simulink model "myrobot"  (R2019b)
settings: Solver=FixedStepAuto  StartTime=0.0  StopTime=2  FixedStep=0.001  MaxStep=0.005  RelTol=1e-3
undefined symbols (not defined in the file or in its folder): X, Y, Z
libraries: sm_lib x17, nesl_utility x13, robotmaniplib x4, simulink x2
(part 1 of 7)
settings Model: Creator=jglee  LastModifiedBy=jglee
settings SolverCC: AlgebraicLoopSolver=LineSearch

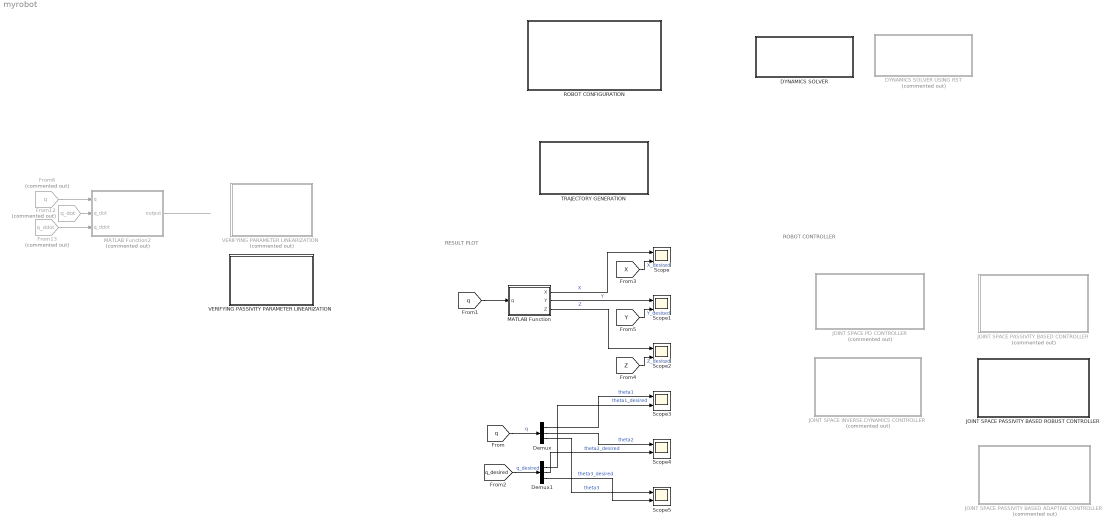
== system myrobot ==
  note: ROBOT CONTROLLER
  note: RESULT PLOT
  DYNAMICS SOLVER : Subsystem
  DYNAMICS SOLVER USING RST : Subsystem  Commented=on
  Demux : Demux  Outputs=3
  Demux1 : Demux  Outputs=3
  From12 : From  Commented=on  GotoTag=q_dot  TagVisibility=global
  From13 : From  Commented=on  GotoTag=q_ddot  TagVisibility=global
  From6 : From  Commented=on  GotoTag=q  TagVisibility=global
  JOINT SPACE INVERSE DYNAMICS CONTROLLER : Subsystem  Commented=on
  JOINT SPACE PASSIVITY BASED ADAPTIVE CONTROLLER : Subsystem  Commented=on
  JOINT SPACE PASSIVITY BASED CONTROLLER : Subsystem  Commented=on
  JOINT SPACE PASSIVITY BASED ROBUST CONTROLLER : Subsystem
  JOINT SPACE PD CONTROLLER : Subsystem  Commented=on
  MATLAB Function : MATLAB Function  TreatAsAtomicUnit=on
  MATLAB Function2 : MATLAB Function  Commented=on  TreatAsAtomicUnit=on
  ROBOT CONFIGURATION : Subsystem
  Scope{,1..5} (6 alike) : Scope  NumInputPorts=2
  TRAJECTORY GENERATION : Subsystem
  VERIFYING PARAMETER LINEARIZATION : Subsystem  Commented=on
  VERIFYING PASSIVITY PARAMETER LINEARIZATION : Subsystem
  wires:
  [q] -> MATLAB Function/1(q)
  MATLAB Function/2(Y) -> Scope1/1  "Y"
  [q] -> Demux/1  "q"
  [q_desired] -> Demux1/1  "q_desired"
  From12/1 -> MATLAB Function2/2(q_dot)
  MATLAB Function2/1(output) -> ?
  From13/1 -> MATLAB Function2/3(q_ddot)
  From6/1 -> MATLAB Function2/1(q)
  [Z] -> Scope2/2  "Z_desired"
  [X] -> Scope/2  "X_desired"
  MATLAB Function/1(X) -> Scope/1  "X"
  [Y] -> Scope1/2  "Y_desired"
  MATLAB Function/3(Z) -> Scope2/1  "Z"
  Demux/1 -> Scope3/1  "theta1"
  Demux/2 -> Scope4/1  "theta2"
  Demux/3 -> Scope5/1  "theta3"
  Demux1/1 -> Scope3/2  "theta1_desired"
  Demux1/2 -> Scope4/2  "theta2_desired"
  Demux1/3 -> Scope5/2  "theta3_desired"

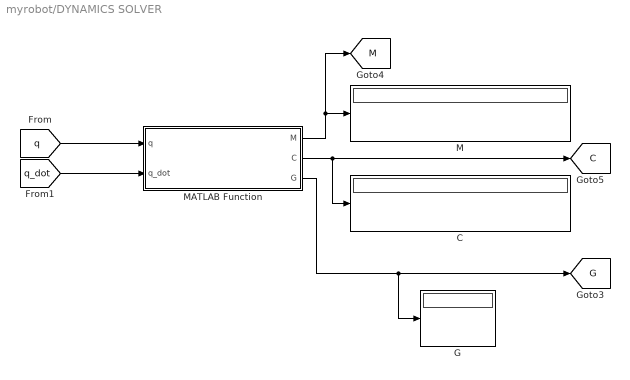
== system myrobot/DYNAMICS SOLVER ==
  C : Display
  G : Display
  M : Display
  MATLAB Function : MATLAB Function  TreatAsAtomicUnit=on
  tag scope: C=global, G=global, M=global
  wires:
  [q] -> MATLAB Function/1(q)
  [q_dot] -> MATLAB Function/2(q_dot)
  MATLAB Function/3(G) -> G/1, [G]
  MATLAB Function/2(C) -> [C], C/1
  MATLAB Function/1(M) -> [M], M/1

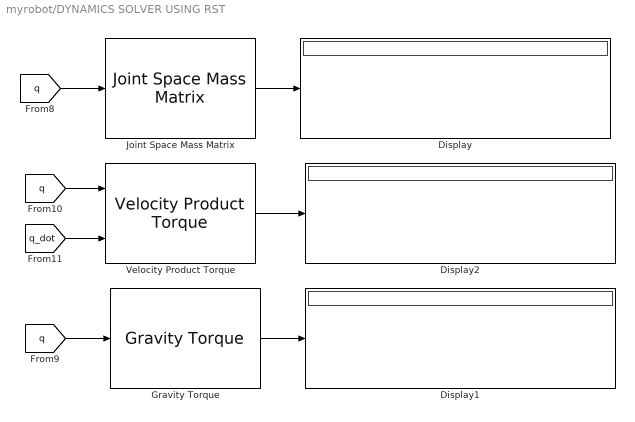
== system myrobot/DYNAMICS SOLVER USING RST ==
  Display : Display
  Display1 : Display
  Display2 : Display
  Gravity Torque : robotmaniplib/Gravity Torque  RigidBodyTree=robot  SimulateUsing=Interpreted execution
      settings: SourceProductName=Robotics System Toolbox
  Joint Space Mass Matrix : robotmaniplib/Joint Space Mass Matrix  RigidBodyTree=robot  SimulateUsing=Interpreted execution
      settings: SourceProductName=Robotics System Toolbox
  Velocity Product Torque : robotmaniplib/Velocity Product Torque  RigidBodyTree=robot  SimulateUsing=Interpreted execution
      settings: SourceProductName=Robotics System Toolbox  SourceProductBaseCode=RO
  wires:
  Joint Space Mass Matrix/1 -> Display/1
  [q_dot] -> Velocity Product Torque/2
  [q] -> Gravity Torque/1
  [q] -> Joint Space Mass Matrix/1
  Velocity Product Torque/1 -> Display2/1
  Gravity Torque/1 -> Display1/1
  [q] -> Velocity Product Torque/1

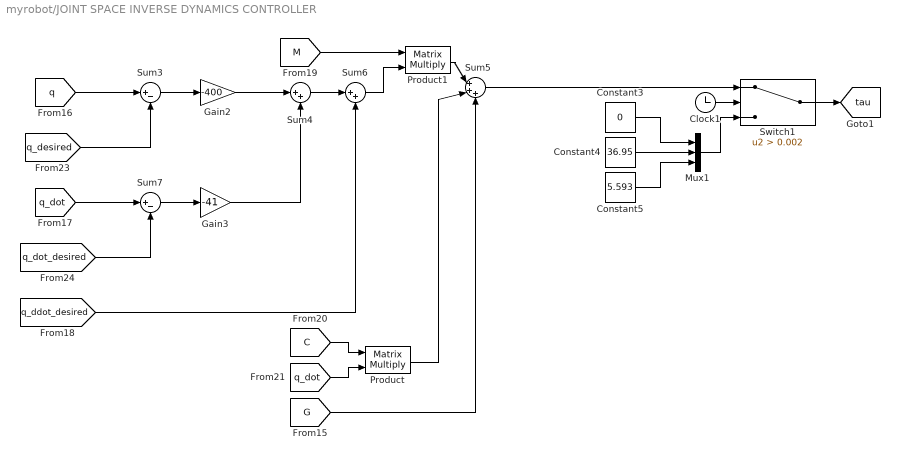
== system myrobot/JOINT SPACE INVERSE DYNAMICS CONTROLLER ==
  Clock1 : Clock
  Constant3 : Constant  Value=0
  Constant4 : Constant  Value=36.95
  Constant5 : Constant  Value=5.593
  Gain2 : Gain  Gain=-400
  Gain3 : Gain  Gain=-41
  Mux1 : Mux  Inputs=3
  Product : Product  Multiplication=Matrix(*)
  Product1 : Product  Multiplication=Matrix(*)
  Sum3 : Sum  Inputs=|+-
  Sum4 : Sum  Inputs=|++
  Sum5 : Sum  Inputs=|+++
  Sum6 : Sum  Inputs=|++
  Sum7 : Sum  Inputs=|+-
  Switch1 : Switch  Criteria=u2 > Threshold  Threshold=0.002
  tag scope: tau=global
  wires:
  Sum5/1 -> Switch1/1
  Sum4/1 -> Sum6/1
  [q_dot_desired] -> Sum7/2
  Mux1/1 -> Switch1/3
  Sum7/1 -> Gain3/1
  [q_desired] -> Sum3/2
  [q] -> Sum3/1
  [q_dot] -> Sum7/1
  Gain3/1 -> Sum4/2
  Product/1 -> Sum5/2
  [G] -> Sum5/3
  Clock1/1 -> Switch1/2
  Product1/1 -> Sum5/1
  [C] -> Product/1
  [M] -> Product1/1
  [q_ddot_desired] -> Sum6/2
  Sum6/1 -> Product1/2
  Gain2/1 -> Sum4/1
  Sum3/1 -> Gain2/1
  [q_dot] -> Product/2
  Constant3/1 -> Mux1/1
  Constant5/1 -> Mux1/3
  Constant4/1 -> Mux1/2
  Switch1/1 -> [tau]

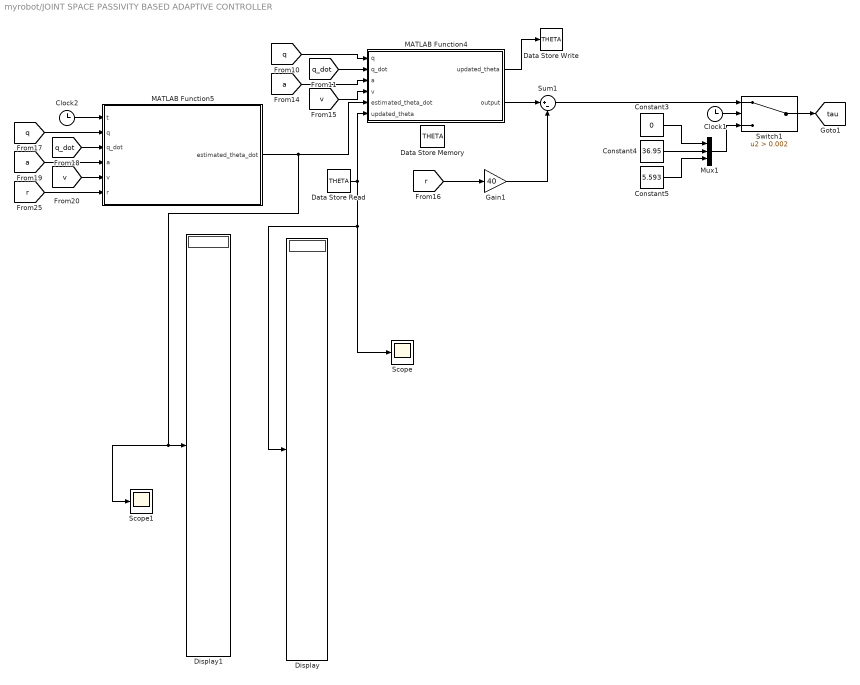
== system myrobot/JOINT SPACE PASSIVITY BASED ADAPTIVE CONTROLLER ==
  Clock1 : Clock
  Clock2 : Clock
  Constant3 : Constant  Value=0
  Constant4 : Constant  Value=36.95
  Constant5 : Constant  Value=5.593
  Data Store Memory : DataStoreMemory  DataStoreName=THETA  ReadBeforeWriteMsg=warning  WriteAfterWriteMsg=warning  WriteAfterReadMsg=warning  InitialValue=[0.253740000000000,1.41285000000000e-07,0.0754340000000000,0.0212824000000000,-7.13886000000000e-08,2.67415000000000e-08,0.00604953000000000,0.00499483000000000,0.0104250000000000,2.13561000000000e-09,0.247523000000000,0.00274946000000000,0.0744749000000000,2.21400980000000,1.73854678600000,0.622883338500000,0.0521152000000000,0.0329527040000000,0.952024214000000,0.000192286280344500,0.371183215904572,0.0688146654633342,0.0753533118750375,0.0294165347194417,0.177120784000000,0.139083742880000,0.0598856414640000,0.0498306670800000,-0.0311344561750400,0.267839835555000,-0.167347701940840,0.159821302798087,-0.0470811354471933]  ShowAdditionalParam=off
  Data Store Read : DataStoreRead  DataStoreName=THETA
  Data Store Write : DataStoreWrite  DataStoreName=THETA
  Display : Display
  Display1 : Display
  Gain1 : Gain  Gain=40
  MATLAB Function4 : MATLAB Function  TreatAsAtomicUnit=on
  MATLAB Function5 : MATLAB Function  TreatAsAtomicUnit=on
  Mux1 : Mux  Inputs=3
  Scope : Scope
  Scope1 : Scope
  Sum1 : Sum  Inputs=|+-
  Switch1 : Switch  Criteria=u2 > Threshold  Threshold=0.002
  tag scope: tau=global
  wires:
  [r] -> Gain1/1
  Clock1/1 -> Switch1/2
  [q] -> MATLAB Function5/2(q)
  [v] -> MATLAB Function4/4(v)
  Constant3/1 -> Mux1/1
  Gain1/1 -> Sum1/2
  [q_dot] -> MATLAB Function5/3(q_dot)
  [r] -> MATLAB Function5/6(r)
  MATLAB Function4/2(output) -> Sum1/1
  [q] -> MATLAB Function4/1(q)
  Mux1/1 -> Switch1/3
  MATLAB Function4/1(updated_theta) -> Data Store Write/1
  [q_dot] -> MATLAB Function4/2(q_dot)
  [a] -> MATLAB Function5/4(a)
  [v] -> MATLAB Function5/5(v)
  Constant4/1 -> Mux1/2
  Data Store Read/1 -> MATLAB Function4/6("updated_theta "), Scope/1, Display/1
  Switch1/1 -> [tau]
  Constant5/1 -> Mux1/3
  [a] -> MATLAB Function4/3(a)
  Sum1/1 -> Switch1/1
  MATLAB Function5/1(estimated_theta_dot) -> Display1/1, Scope1/1, MATLAB Function4/5(estimated_theta_dot)
  Clock2/1 -> MATLAB Function5/1(t)

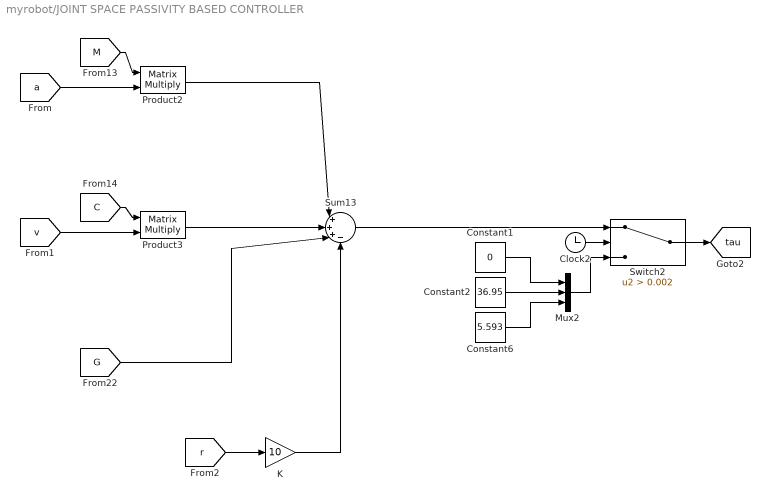
== system myrobot/JOINT SPACE PASSIVITY BASED CONTROLLER ==
  Clock2 : Clock
  Constant1 : Constant  Value=0
  Constant2 : Constant  Value=36.95
  Constant6 : Constant  Value=5.593
  "K " : Gain  Gain=10
  Mux2 : Mux  Inputs=3
  Product2 : Product  Multiplication=Matrix(*)
  Product3 : Product  Multiplication=Matrix(*)
  Sum13 : Sum  Inputs=|+++-
  Switch2 : Switch  Criteria=u2 > Threshold  Threshold=0.002
  tag scope: tau=global
  wires:
  [a] -> Product2/2
  [v] -> Product3/2
  [r] -> "K "/1
  "K "/1 -> Sum13/4
  Clock2/1 -> Switch2/2
  [M] -> Product2/1
  [G] -> Sum13/3
  Mux2/1 -> Switch2/3
  Sum13/1 -> Switch2/1
  Product3/1 -> Sum13/2
  Constant6/1 -> Mux2/3
  Constant2/1 -> Mux2/2
  Switch2/1 -> [tau]
  Constant1/1 -> Mux2/1
  [C] -> Product3/1
  Product2/1 -> Sum13/1

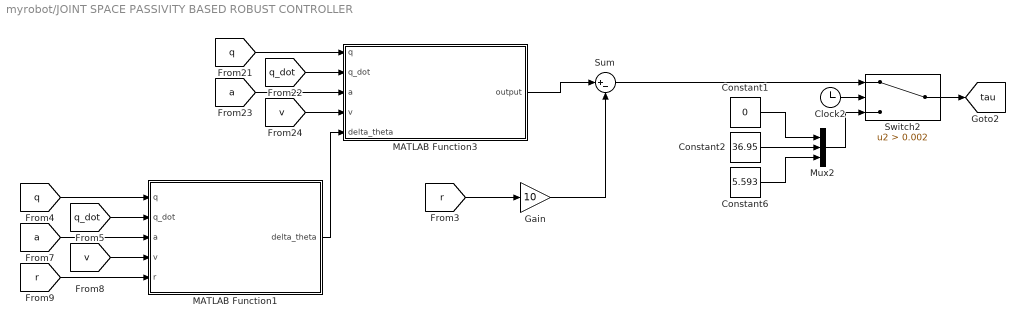
== system myrobot/JOINT SPACE PASSIVITY BASED ROBUST CONTROLLER ==
  Clock2 : Clock
  Constant1 : Constant  Value=0
  Constant2 : Constant  Value=36.95
  Constant6 : Constant  Value=5.593
  Gain : Gain  Gain=10
  MATLAB Function1 : MATLAB Function  TreatAsAtomicUnit=on
  MATLAB Function3 : MATLAB Function  TreatAsAtomicUnit=on
  Mux2 : Mux  Inputs=3
  Sum : Sum  Inputs=|+-
  Switch2 : Switch  Criteria=u2 > Threshold  Threshold=0.002
  tag scope: tau=global
  wires:
  Gain/1 -> Sum/2
  MATLAB Function3/1(output) -> Sum/1
  Sum/1 -> Switch2/1
  MATLAB Function1/1(delta_theta) -> MATLAB Function3/5(delta_theta)
  [q] -> MATLAB Function1/1(q)
  [a] -> MATLAB Function3/3(a)
  Mux2/1 -> Switch2/3
  [a] -> MATLAB Function1/3(a)
  [q_dot] -> MATLAB Function1/2(q_dot)
  [r] -> MATLAB Function1/5(r)
  [q] -> MATLAB Function3/1(q)
  Switch2/1 -> [tau]
  Clock2/1 -> Switch2/2
  Constant6/1 -> Mux2/3
  [v] -> MATLAB Function1/4(v)
  Constant2/1 -> Mux2/2
  Constant1/1 -> Mux2/1
  [q_dot] -> MATLAB Function3/2(q_dot)
  [v] -> MATLAB Function3/4(v)
  [r] -> Gain/1

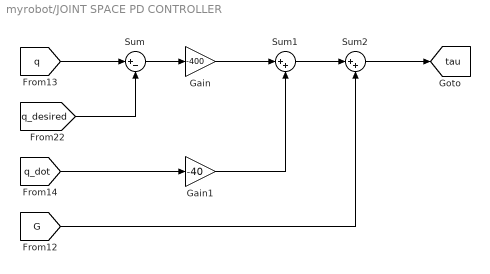
== system myrobot/JOINT SPACE PD CONTROLLER ==
  Gain : Gain  Gain=-400
  Gain1 : Gain  Gain=-40
  Sum : Sum  Inputs=|+-
  Sum1 : Sum  Inputs=|++
  Sum2 : Sum  Inputs=|++
  tag scope: tau=global
  wires:
  [q_desired] -> Sum/2
  Gain/1 -> Sum1/1
  Sum2/1 -> [tau]
  Sum/1 -> Gain/1
  [q_dot] -> Gain1/1
  Gain1/1 -> Sum1/2
  [q] -> Sum/1
  Sum1/1 -> Sum2/1
  [G] -> Sum2/2

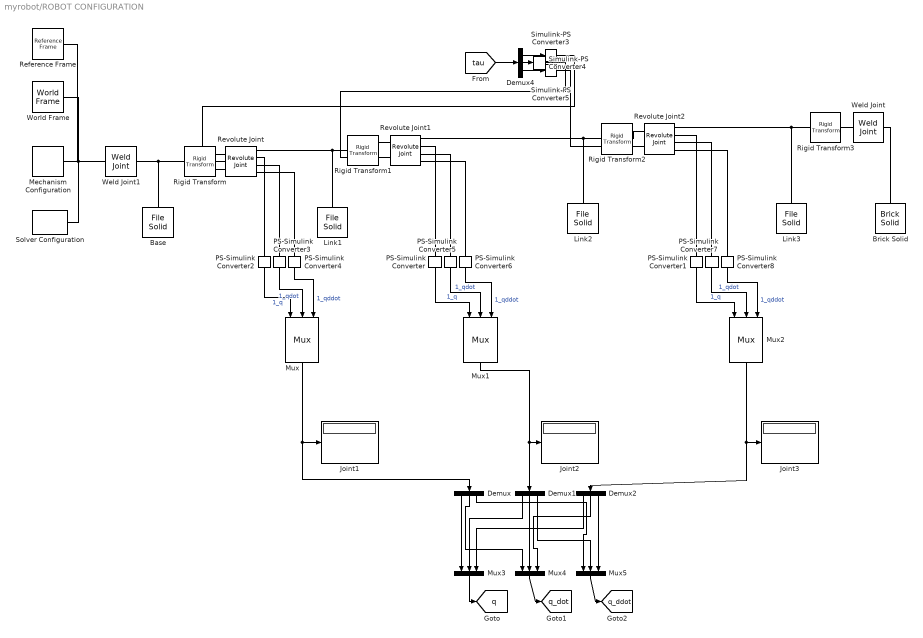
== system myrobot/ROBOT CONFIGURATION ==
  Base : sm_lib/Body Elements/File Solid  ExtGeomFileName=Base.ipt  UnitType=FromFile  ExtGeomFileUnits=m  StepReaderType=HEX  ExportEntireGeometry=off  InertiaType=CalculateFromGeometry  Mass=1  MassUnits=kg  CenterOfMass=[0 0 0]  CenterOfMassUnits=m  MomentsOfInertia=[1 1 1]  MomentsOfInertiaUnits=kg*m^2  ProductsOfInertia=[0 0 0]  ProductsOfInertiaUnits=kg*m^2  BasedOnType=Density  Density=1.06  DensityUnits=g/cm^3  DoExposeReferenceFrame=on  SerializedFrames=<Frames/>  GraphicType=FromGeometry  MarkerShape=Sphere  MarkerSize=10  GraphicVisPropType=FromFileVisualProperties  GraphicDiffuseColor=[0.5 0.5 0.5]  GraphicSpecularColor=[0.5 0.5 0.5 1.0]  GraphicAmbientColor=[0.15 0.15 0.15 1.0]  GraphicEmissiveColor=[0.0 0.0 0.0 1.0]  GraphicShininess=75  GraphicOpacity=1.0
  Brick Solid : sm_lib/Body Elements/Brick Solid  GraphicAmbientColor=[0.15 0.15 0.15 1.0]  BasedOnType=Density  BrickDimensions=[1 1 1]  BrickDimensionUnits=cm  CenterOfMass=[0 0 0]  CenterOfMassUnits=m  GraphicDiffuseColor=[0.5 0.5 0.5]  Density=2000  DensityUnits=g/cm^3  DoExposeReferenceFrame=on  GraphicEmissiveColor=[0.0 0.0 0.0 1.0]  ExportEntireGeometry=off  SerializedFrames=<Frames/>  MarkerShape=Sphere  MarkerSize=10  GraphicType=FromGeometry  InertiaType=CalculateFromGeometry  Mass=1  MassUnits=kg  MomentsOfInertia=[1 1 1]  MomentsOfInertiaUnits=kg*m^2  GraphicOpacity=1.0  ProductsOfInertia=[0 0 0]  ProductsOfInertiaUnits=kg*m^2  GraphicShininess=75  GraphicSpecularColor=[0.5 0.5 0.5 1.0]  GraphicVisPropType=SimpleVisualProperties
  Demux{,1..2,4} (4 alike) : Demux  Outputs=3
  Joint1 : Display
  Joint2 : Display
  Joint3 : Display
  "Link1 " : sm_lib/Body Elements/File Solid  ExtGeomFileName=Link1.ipt  UnitType=FromFile  ExtGeomFileUnits=m  StepReaderType=HEX  ExportEntireGeometry=off  InertiaType=CalculateFromGeometry  Mass=1  MassUnits=kg  CenterOfMass=[0 0 0]  CenterOfMassUnits=m  MomentsOfInertia=[1 1 1]  MomentsOfInertiaUnits=kg*m^2  ProductsOfInertia=[0 0 0]  ProductsOfInertiaUnits=kg*m^2  BasedOnType=Density  Density=1.06  DensityUnits=g/cm^3  DoExposeReferenceFrame=on  SerializedFrames=<Frames/>  GraphicType=FromGeometry  MarkerShape=Sphere  MarkerSize=10  GraphicVisPropType=SimpleVisualProperties  GraphicDiffuseColor=[0.5 0.5 0.5]  GraphicSpecularColor=[0.5 0.5 0.5 1.0]  GraphicAmbientColor=[0.15 0.15 0.15 1.0]  GraphicEmissiveColor=[0.0 0.0 0.0 1.0]  GraphicShininess=75  GraphicOpacity=1.0
  "Link2 " : sm_lib/Body Elements/File Solid  ExtGeomFileName=Link2.ipt  UnitType=FromFile  ExtGeomFileUnits=m  StepReaderType=HEX  ExportEntireGeometry=off  InertiaType=CalculateFromGeometry  Mass=1  MassUnits=kg  CenterOfMass=[0 0 0]  CenterOfMassUnits=m  MomentsOfInertia=[1 1 1]  MomentsOfInertiaUnits=kg*m^2  ProductsOfInertia=[0 0 0]  ProductsOfInertiaUnits=kg*m^2  BasedOnType=Density  Density=1.06  DensityUnits=g/cm^3  DoExposeReferenceFrame=on  SerializedFrames=<Frames/>  GraphicType=FromGeometry  MarkerShape=Sphere  MarkerSize=10  GraphicVisPropType=SimpleVisualProperties  GraphicDiffuseColor=[0.5 0.5 0.5]  GraphicSpecularColor=[0.5 0.5 0.5 1.0]  GraphicAmbientColor=[0.15 0.15 0.15 1.0]  GraphicEmissiveColor=[0.0 0.0 0.0 1.0]  GraphicShininess=75  GraphicOpacity=1.0
  Link3 : sm_lib/Body Elements/File Solid  ExtGeomFileName=Link3.ipt  UnitType=FromFile  ExtGeomFileUnits=m  StepReaderType=HEX  ExportEntireGeometry=off  InertiaType=CalculateFromGeometry  Mass=1  MassUnits=kg  CenterOfMass=[0 0 0]  CenterOfMassUnits=m  MomentsOfInertia=[1 1 1]  MomentsOfInertiaUnits=kg*m^2  ProductsOfInertia=[0 0 0]  ProductsOfInertiaUnits=kg*m^2  BasedOnType=Density  Density=1.06  DensityUnits=g/cm^3  DoExposeReferenceFrame=on  SerializedFrames=<Frames/>  GraphicType=FromGeometry  MarkerShape=Sphere  MarkerSize=10  GraphicVisPropType=SimpleVisualProperties  GraphicDiffuseColor=[0.5 0.5 0.5]  GraphicSpecularColor=[0.5 0.5 0.5 1.0]  GraphicAmbientColor=[0.15 0.15 0.15 1.0]  GraphicEmissiveColor=[0.0 0.0 0.0 1.0]  GraphicShininess=75  GraphicOpacity=1.0
  Mechanism Configuration : sm_lib/Utilities/Mechanism Configuration  UniformGravity=Constant  GravityVector=[0 0 -9.81]  GravityUnits=m/s^2  LinearizationDelta=0.001
  Mux{,1..5} (6 alike) : Mux  Inputs=3
      Mux settings: DisplayOption=signals
      Mux1 settings: DisplayOption=signals
      Mux2 settings: DisplayOption=signals
  PS-Simulink Converter{,1..8} (9 alike) : nesl_utility/PS-Simulink Converter  PhysicalDomain=network_engine_domain  SubClassName=ps_output  LeftPortType=input  RightPortType=output  PseudoPeriodic=off  Frequencies=[]  Unit=inherit  AffineConversion=off
  Reference Frame : sm_lib/Frames and Transforms/Reference Frame
  Revolute Joint : sm_lib/Joints/Revolute Joint  JointMode=Normal  SenseConstraintForce=off  SenseConstraintForceX=off  SenseConstraintForceY=off  SenseConstraintForceZ=off  SenseConstraintTorque=off  SenseConstraintTorqueX=off  SenseConstraintTorqueY=off  SenseConstraintTorqueZ=off  SenseTotalForce=off  SenseTotalForceX=off  SenseTotalForceY=off  SenseTotalForceZ=off  SenseTotalTorque=off  SenseTotalTorqueX=off  SenseTotalTorqueY=off  SenseTotalTorqueZ=off  CompositeWrenchDir=FollowerOnBase  CompositeWrenchFrame=BaseFrame  EquilibriumPosition=0  EquilibriumPositionUnits=deg  SpringStiffness=0  SpringStiffnessUnits=N*m/deg  DampingCoefficient=0.0  DampingCoefficientUnits=N*m/(deg/s)  TorqueActuationMode=InputTorque  MotionActuationMode=ComputedMotion  SensePosition=on  SenseVelocity=on  SenseAcceleration=on  SenseTorqueForce=off  SenseLowerLimitTorqueForce=off  SenseUpperLimitTorqueForce=off  LowerLimitSpecify=off  LowerLimitBound=-90  LowerLimitBoundUnits=deg  LowerLimitStiffness=1e4  LowerLimitStiffnessUnits=N*m/deg  LowerLimitDamping=10  LowerLimitDampingUnits=N*m/(deg/s)  LowerLimitTransitionRegionWidth=0.1  LowerLimitTransitionRegionWidthUnits=deg  UpperLimitSpecify=off  UpperLimitBound=90  UpperLimitBoundUnits=deg  UpperLimitStiffness=1e4  UpperLimitStiffnessUnits=N*m/deg  UpperLimitDamping=10  UpperLimitDampingUnits=N*m/(deg/s)  UpperLimitTransitionRegionWidth=0.1  UpperLimitTransitionRegionWidthUnits=deg  PositionTargetSpecify=on  PositionTargetPriority=High  PositionTargetValue=-0.838  PositionTargetValueUnits=rad  VelocityTargetSpecify=off  VelocityTargetPriority=High  VelocityTargetValue=0  VelocityTargetValueUnits=deg/s
  Revolute Joint1 : sm_lib/Joints/Revolute Joint  JointMode=Normal  SenseConstraintForce=off  SenseConstraintForceX=off  SenseConstraintForceY=off  SenseConstraintForceZ=off  SenseConstraintTorque=off  SenseConstraintTorqueX=off  SenseConstraintTorqueY=off  SenseConstraintTorqueZ=off  SenseTotalForce=off  SenseTotalForceX=off  SenseTotalForceY=off  SenseTotalForceZ=off  SenseTotalTorque=off  SenseTotalTorqueX=off  SenseTotalTorqueY=off  SenseTotalTorqueZ=off  CompositeWrenchDir=FollowerOnBase  CompositeWrenchFrame=BaseFrame  EquilibriumPosition=0  EquilibriumPositionUnits=deg  SpringStiffness=0  SpringStiffnessUnits=N*m/deg  DampingCoefficient=0.0  DampingCoefficientUnits=N*m/(deg/s)  TorqueActuationMode=InputTorque  MotionActuationMode=ComputedMotion  SensePosition=on  SenseVelocity=on  SenseAcceleration=on  SenseTorqueForce=off  SenseLowerLimitTorqueForce=off  SenseUpperLimitTorqueForce=off  LowerLimitSpecify=off  LowerLimitBound=-90  LowerLimitBoundUnits=deg  LowerLimitStiffness=1e4  LowerLimitStiffnessUnits=N*m/deg  LowerLimitDamping=10  LowerLimitDampingUnits=N*m/(deg/s)  LowerLimitTransitionRegionWidth=0.1  LowerLimitTransitionRegionWidthUnits=deg  UpperLimitSpecify=off  UpperLimitBound=90  UpperLimitBoundUnits=deg  UpperLimitStiffness=1e4  UpperLimitStiffnessUnits=N*m/deg  UpperLimitDamping=10  UpperLimitDampingUnits=N*m/(deg/s)  UpperLimitTransitionRegionWidth=0.1  UpperLimitTransitionRegionWidthUnits=deg  PositionTargetSpecify=on  PositionTargetPriority=High  PositionTargetValue=-0.9973  PositionTargetValueUnits=rad  VelocityTargetSpecify=off  VelocityTargetPriority=High  VelocityTargetValue=0  VelocityTargetValueUnits=deg/s
  Revolute Joint2 : sm_lib/Joints/Revolute Joint  JointMode=Normal  SenseConstraintForce=off  SenseConstraintForceX=off  SenseConstraintForceY=off  SenseConstraintForceZ=off  SenseConstraintTorque=off  SenseConstraintTorqueX=off  SenseConstraintTorqueY=off  SenseConstraintTorqueZ=off  SenseTotalForce=off  SenseTotalForceX=off  SenseTotalForceY=off  SenseTotalForceZ=off  SenseTotalTorque=off  SenseTotalTorqueX=off  SenseTotalTorqueY=off  SenseTotalTorqueZ=off  CompositeWrenchDir=FollowerOnBase  CompositeWrenchFrame=BaseFrame  EquilibriumPosition=0  EquilibriumPositionUnits=deg  SpringStiffness=0  SpringStiffnessUnits=N*m/deg  DampingCoefficient=0.0  DampingCoefficientUnits=N*m/(deg/s)  TorqueActuationMode=InputTorque  MotionActuationMode=ComputedMotion  SensePosition=on  SenseVelocity=on  SenseAcceleration=on  SenseTorqueForce=off  SenseLowerLimitTorqueForce=off  SenseUpperLimitTorqueForce=off  LowerLimitSpecify=off  LowerLimitBound=-90  LowerLimitBoundUnits=deg  LowerLimitStiffness=1e4  LowerLimitStiffnessUnits=N*m/deg  LowerLimitDamping=10  LowerLimitDampingUnits=N*m/(deg/s)  LowerLimitTransitionRegionWidth=0.1  LowerLimitTransitionRegionWidthUnits=deg  UpperLimitSpecify=off  UpperLimitBound=90  UpperLimitBoundUnits=deg  UpperLimitStiffness=1e4  UpperLimitStiffnessUnits=N*m/deg  UpperLimitDamping=10  UpperLimitDampingUnits=N*m/(deg/s)  UpperLimitTransitionRegionWidth=0.1  UpperLimitTransitionRegionWidthUnits=deg  PositionTargetSpecify=on  PositionTargetPriority=High  PositionTargetValue=-0.9505  PositionTargetValueUnits=rad  VelocityTargetSpecify=off  VelocityTargetPriority=High  VelocityTargetValue=0  VelocityTargetValueUnits=deg/s
  Rigid Transform : sm_lib/Frames and Transforms/Rigid Transform  TranslationMethod=Cartesian  TranslationStandardOffset=0  TranslationLengthUnit=m  TranslationStandardAxis=+Z  TranslationCartesianOffset=[0 0 0.07]  TranslationROffset=0  TranslationROffsetUnits=m  TranslationZOffset=0  TranslationZOffsetUnits=m  TranslationThetaOffset=0  TranslationThetaOffsetUnits=deg  RotationMethod=RotationMatrix  RotationAngleUnits=deg  RotationStandardAxis=+Z  RotationAngle=0.0  RotationArbitraryAxis=[0 0 1]  FollAlignAxisA=+X  BaseAlignAxisA=+Y  FollAlignAxisB=+Y  BaseAlignAxisB=+Z  RotationSequenceAxes=FollowerAxes  RotationSequence=XYX  RotationSequenceAngles=[0 0 0]  RotationSequenceAnglesUnits=deg  RotationMatrix=[1 0 0; 0 1 0; 0 0 1]
  Rigid Transform1 : sm_lib/Frames and Transforms/Rigid Transform  TranslationMethod=Cartesian  TranslationStandardOffset=0  TranslationLengthUnit=m  TranslationStandardAxis=+Z  TranslationCartesianOffset=[0.08 0 0.12]  TranslationROffset=0  TranslationROffsetUnits=m  TranslationZOffset=0  TranslationZOffsetUnits=m  TranslationThetaOffset=0  TranslationThetaOffsetUnits=deg  RotationMethod=RotationMatrix  RotationAngleUnits=deg  RotationStandardAxis=+Z  RotationAngle=0.0  RotationArbitraryAxis=[0 0 1]  FollAlignAxisA=+X  BaseAlignAxisA=+Y  FollAlignAxisB=+Y  BaseAlignAxisB=+Z  RotationSequenceAxes=FollowerAxes  RotationSequence=XYX  RotationSequenceAngles=[0 0 0]  RotationSequenceAnglesUnits=deg  RotationMatrix=[0 0 1; 1 0 0; 0 1 0]
  Rigid Transform2 : sm_lib/Frames and Transforms/Rigid Transform  TranslationMethod=Cartesian  TranslationStandardOffset=0  TranslationLengthUnit=m  TranslationStandardAxis=+Z  TranslationCartesianOffset=[0 0.43 0]  TranslationROffset=0  TranslationROffsetUnits=m  TranslationZOffset=0  TranslationZOffsetUnits=m  TranslationThetaOffset=0  TranslationThetaOffsetUnits=deg  RotationMethod=RotationMatrix  RotationAngleUnits=deg  RotationStandardAxis=+Z  RotationAngle=0.0  RotationArbitraryAxis=[0 0 1]  FollAlignAxisA=+X  BaseAlignAxisA=+Y  FollAlignAxisB=+Y  BaseAlignAxisB=+Z  RotationSequenceAxes=FollowerAxes  RotationSequence=XYX  RotationSequenceAngles=[0 0 0]  RotationSequenceAnglesUnits=deg  RotationMatrix=[1 0 0; 0 1 0; 0 0 1]
  Rigid Transform3 : sm_lib/Frames and Transforms/Rigid Transform  TranslationMethod=Cartesian  TranslationStandardOffset=0  TranslationLengthUnit=m  TranslationStandardAxis=+Z  TranslationCartesianOffset=[0 0.335 -0.08]  TranslationROffset=0  TranslationROffsetUnits=m  TranslationZOffset=0  TranslationZOffsetUnits=m  TranslationThetaOffset=0  TranslationThetaOffsetUnits=deg  RotationMethod=None  RotationAngleUnits=deg  RotationStandardAxis=+Z  RotationAngle=0.0  RotationArbitraryAxis=[0 0 1]  FollAlignAxisA=+X  BaseAlignAxisA=+Y  FollAlignAxisB=+Y  BaseAlignAxisB=+Z  RotationSequenceAxes=FollowerAxes  RotationSequence=XYX  RotationSequenceAngles=[0 0 0]  RotationSequenceAnglesUnits=deg  RotationMatrix=[1 0 0; 0 1 0; 0 0 1]
  Simulink-PS Converter3 : nesl_utility/Simulink-PS Converter  PhysicalDomain=network_engine_domain  SubClassName=ps_input  LeftPortType=input  RightPortType=output  PseudoPeriodic=off  Frequencies=[]  NoiseDistribution=none  NoiseParameters=[]  Unit=1  AffineConversion=off  FilteringAndDerivatives=filter  SimscapeFilterOrder=2  InputFilterTimeConstant=0.005  UdotUserProvided=0
  Simulink-PS Converter4 : nesl_utility/Simulink-PS Converter  PhysicalDomain=network_engine_domain  SubClassName=ps_input  LeftPortType=input  RightPortType=output  PseudoPeriodic=off  Frequencies=[]  NoiseDistribution=none  NoiseParameters=[]  Unit=1  AffineConversion=off  FilteringAndDerivatives=filter  SimscapeFilterOrder=2  InputFilterTimeConstant=0.005  UdotUserProvided=0
  Simulink-PS Converter5 : nesl_utility/Simulink-PS Converter  PhysicalDomain=network_engine_domain  SubClassName=ps_input  LeftPortType=input  RightPortType=output  PseudoPeriodic=off  Frequencies=[]  NoiseDistribution=none  NoiseParameters=[]  Unit=1  AffineConversion=off  FilteringAndDerivatives=filter  SimscapeFilterOrder=2  InputFilterTimeConstant=0.005  UdotUserProvided=0
  Solver Configuration : nesl_utility/Solver Configuration  PhysicalDomain=network_engine_domain  SubClassName=solver  LeftPortType=input  RightPortType=generic  Tones=[]  Harmonics=[]  SimulateNoise=off  Profile=off  UseLocalSampling=off  EnableSwitchedLinearOptims=on  FrequencyDomain=off  UseCCode=off  RelTol=0.001  AbsTol=1e-06  MinStep=1e-09  ToWorkspace=off  RevertToSquareIcSolve=off  NumHomotopyIterations=100  PhasorMode=off  PhasorModeNumHarmonics=1  DoDC=off  ResidualTolerance=1e-09  UseLocalSolver=off  LocalSolverChoice=NE_BACKWARD_EULER_ADVANCER  LocalSolverSampleTime=0.001  DoFixedCost=off  MaxNonlinIter=3  MaxModeIter=2  LinearAlgebra=auto  EquationFormulation=NE_TIME_EF  DelaysMemoryBudget=1024  AutomaticFiltering=on  FilteringTimeConstant=0.001  PartitionStorageMethod=AS_NEEDED  PartitionMemoryBudget=1024  PartitionMethod=ROBUST
  Weld Joint : sm_lib/Joints/Weld Joint  JointMode=Normal  SenseConstraintForce=off  SenseConstraintForceX=off  SenseConstraintForceY=off  SenseConstraintForceZ=off  SenseConstraintTorque=off  SenseConstraintTorqueX=off  SenseConstraintTorqueY=off  SenseConstraintTorqueZ=off  SenseTotalForce=off  SenseTotalForceX=off  SenseTotalForceY=off  SenseTotalForceZ=off  SenseTotalTorque=off  SenseTotalTorqueX=off  SenseTotalTorqueY=off  SenseTotalTorqueZ=off  CompositeWrenchDir=FollowerOnBase  CompositeWrenchFrame=BaseFrame
  Weld Joint1 : sm_lib/Joints/Weld Joint  JointMode=Normal  SenseConstraintForce=off  SenseConstraintForceX=off  SenseConstraintForceY=off  SenseConstraintForceZ=off  SenseConstraintTorque=off  SenseConstraintTorqueX=off  SenseConstraintTorqueY=off  SenseConstraintTorqueZ=off  SenseTotalForce=off  SenseTotalForceX=off  SenseTotalForceY=off  SenseTotalForceZ=off  SenseTotalTorque=off  SenseTotalTorqueX=off  SenseTotalTorqueY=off  SenseTotalTorqueZ=off  CompositeWrenchDir=FollowerOnBase  CompositeWrenchFrame=BaseFrame
  World Frame : sm_lib/Frames and Transforms/World Frame
  tag scope: q=global, q_ddot=global, q_dot=global
  wires:
  Demux1/1 -> Mux3/2
  Demux/3 -> Mux5/1
  Mux3/1 -> [q]
  Mux2/1 -> Joint3/1, Demux2/1
  Demux2/3 -> Mux5/3
  PS-Simulink Converter8/1 -> Mux2/3  "1_qddot"
  Demux/1 -> Mux3/1
  PS-Simulink Converter2/1 -> Mux/1  "1_q"
  PS-Simulink Converter5/1 -> Mux1/2  "1_qdot"
  PS-Simulink Converter7/1 -> Mux2/2  "1_qdot"
  PS-Simulink Converter4/1 -> Mux/3  "1_qddot"
  PS-Simulink Converter3/1 -> Mux/2  "1_qdot"
  PS-Simulink Converter/1 -> Mux1/1  "1_q"
  Mux/1 -> Demux/1, Joint1/1
  Demux2/1 -> Mux3/3
  Demux/2 -> Mux4/1
  PS-Simulink Converter1/1 -> Mux2/1  "1_q"
  PS-Simulink Converter6/1 -> Mux1/3  "1_qddot"
  Demux1/3 -> Mux5/2
  Mux1/1 -> Joint2/1, Demux1/1
  Mux4/1 -> [q_dot]
  Demux1/2 -> Mux4/2
  Demux2/2 -> Mux4/3
  Mux5/1 -> [q_ddot]
  Demux4/1 -> Simulink-PS Converter3/1
  Demux4/3 -> Simulink-PS Converter5/1
  [tau] -> Demux4/1
  Demux4/2 -> Simulink-PS Converter4/1
  connections:
  Rigid Transform/RConn1 -- Revolute Joint/LConn1
  PS-Simulink Converter3/LConn1 -- Revolute Joint/RConn3
  Revolute Joint2/RConn2 -- PS-Simulink Converter1/LConn1
  "Link2 "/RConn1 -- Rigid Transform2/LConn1 -- Revolute Joint1/RConn1
  Revolute Joint1/RConn2 -- PS-Simulink Converter/LConn1
  PS-Simulink Converter2/LConn1 -- Revolute Joint/RConn2
  PS-Simulink Converter5/LConn1 -- Revolute Joint1/RConn3
  PS-Simulink Converter7/LConn1 -- Revolute Joint2/RConn3
  PS-Simulink Converter8/LConn1 -- Revolute Joint2/RConn4
  Rigid Transform1/LConn1 -- Revolute Joint/RConn1 -- "Link1 "/RConn1
  Revolute Joint2/LConn1 -- Rigid Transform2/RConn1
  Mechanism Configuration/RConn1 -- Weld Joint1/LConn1 -- Reference Frame/RConn1 -- World Frame/RConn1 -- Solver Configuration/RConn1
  Revolute Joint1/LConn1 -- Rigid Transform1/RConn1
  PS-Simulink Converter6/LConn1 -- Revolute Joint1/RConn4
  PS-Simulink Converter4/LConn1 -- Revolute Joint/RConn4
  Link3/RConn1 -- Rigid Transform3/LConn1 -- Revolute Joint2/RConn1
  Simulink-PS Converter3/RConn1 -- Revolute Joint/LConn2
  Simulink-PS Converter4/RConn1 -- Revolute Joint1/LConn2
  Simulink-PS Converter5/RConn1 -- Revolute Joint2/LConn2
  Weld Joint/LConn1 -- Rigid Transform3/RConn1
  Brick Solid/RConn1 -- Weld Joint/RConn1
  Base/RConn1 -- Rigid Transform/LConn1 -- Weld Joint1/RConn1

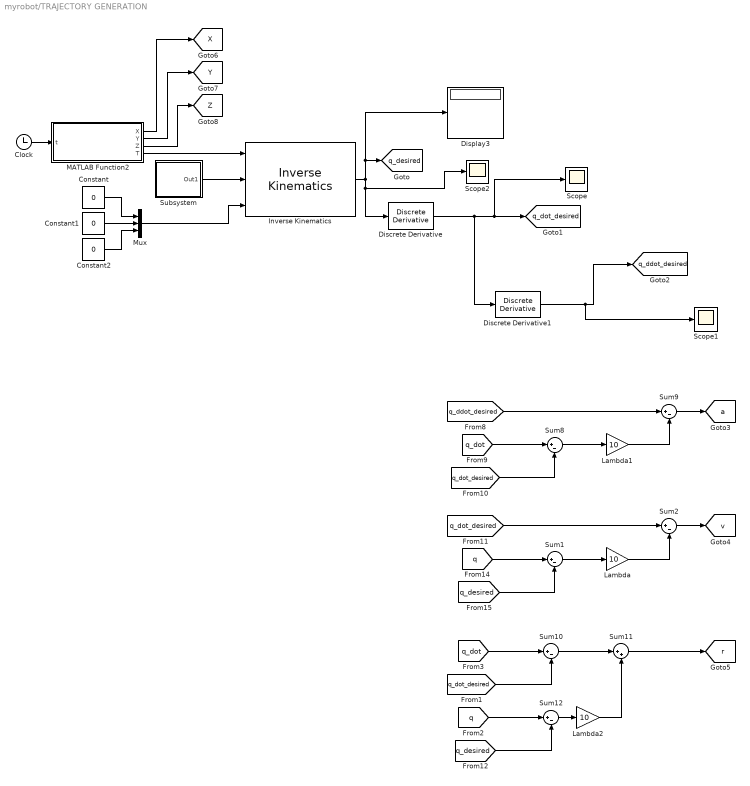
== system myrobot/TRAJECTORY GENERATION ==
  Clock : Clock
  Constant : Constant  Value=0
  Constant1 : Constant  Value=0
  Constant2 : Constant  Value=0
  Discrete Derivative : simulink/Discrete/Discrete Derivative  gainval=1.0  ICPrevScaledInput=0.0  OutMin=[]  OutMax=[]  OutDataType=fixdt(1, 16)  OutScaling=2^-10  DoSatur=off
  Discrete Derivative1 : simulink/Discrete/Discrete Derivative  gainval=1.0  ICPrevScaledInput=0.0  OutMin=[]  OutMax=[]  OutDataType=fixdt(1, 16)  OutScaling=2^-10  DoSatur=off
  Display3 : Display
  Inverse Kinematics : robotmaniplib/Inverse Kinematics  RigidBodyTree=robot  EndEffector=Body5  ShowInfo=off  SolverName=BFGS Gradient Projection  EnforceJointLimits=on  MaxIterations=1500  MaxTime=10  GradientTolerance=1e-7  SolutionTolerance=1e-6  StepTolerance=1e-14  ErrorChangeTolerance=1e-12  UseErrorDamping=on  DampingBias=0.0025  SimulateUsing=Code generation
      settings: SourceProductName=Robotics System Toolbox
  Lambda : Gain  Gain=10
  Lambda1 : Gain  Gain=10
  Lambda2 : Gain  Gain=10
  MATLAB Function2 : MATLAB Function  TreatAsAtomicUnit=on
  Mux : Mux  Inputs=3
  Scope : Scope
  Scope1 : Scope
  Scope2 : Scope
  Subsystem : Subsystem
  Sum{1..2,8..10,12} (6 alike) : Sum  Inputs=|+-
  Sum11 : Sum  Inputs=|++
  tag scope: X=global, Y=global, Z=global, a=global, q_ddot_desired=global, q_desired=global, q_dot_desired=global, r=global, v=global
  wires:
  Subsystem/1(Out1) -> Inverse Kinematics/2
  Clock/1 -> MATLAB Function2/1(t)
  MATLAB Function2/4(T) -> Inverse Kinematics/1
  Constant/1 -> Mux/1
  Constant1/1 -> Mux/2
  Constant2/1 -> Mux/3
  Mux/1 -> Inverse Kinematics/3
  Inverse Kinematics/1 -> Discrete Derivative/1, Scope2/1, Display3/1, [q_desired]
  Discrete Derivative/1 -> Discrete Derivative1/1, Scope/1, [q_dot_desired]
  Discrete Derivative1/1 -> Scope1/1, [q_ddot_desired]
  Sum9/1 -> [a]
  [q_desired] -> Sum1/2
  [q_dot] -> Sum8/1
  Lambda1/1 -> Sum9/2
  Lambda/1 -> Sum2/2
  [q_dot_desired] -> Sum2/1
  Sum2/1 -> [v]
  Sum8/1 -> Lambda1/1
  Sum1/1 -> Lambda/1
  [q_dot_desired] -> Sum8/2
  [q_ddot_desired] -> Sum9/1
  [q] -> Sum1/1
  [q_desired] -> Sum12/2
  Sum12/1 -> Lambda2/1
  [q_dot_desired] -> Sum10/2
  Sum10/1 -> Sum11/1
  [q_dot] -> Sum10/1
  [q] -> Sum12/1
  Lambda2/1 -> Sum11/2
  Sum11/1 -> [r]
  MATLAB Function2/1(X) -> [X]
  MATLAB Function2/2(Y) -> [Y]
  MATLAB Function2/3(Z) -> [Z]

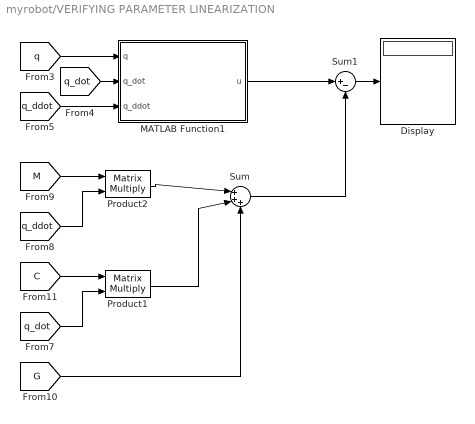
== system myrobot/VERIFYING PARAMETER LINEARIZATION ==
  Display : Display
  MATLAB Function1 : MATLAB Function  TreatAsAtomicUnit=on
  Product1 : Product  Multiplication=Matrix(*)
  Product2 : Product  Multiplication=Matrix(*)
  Sum : Sum  Inputs=|+++
  Sum1 : Sum  Inputs=|+-
  wires:
  Product2/1 -> Sum/1
  [q_dot] -> MATLAB Function1/2(q_dot)
  [q_ddot] -> Product2/2
  [q] -> MATLAB Function1/1(q)
  Product1/1 -> Sum/2
  [C] -> Product1/1
  [G] -> Sum/3
  [q_dot] -> Product1/2
  Sum1/1 -> Display/1
  [M] -> Product2/1
  [q_ddot] -> MATLAB Function1/3(q_ddot)
  MATLAB Function1/1(u) -> Sum1/1
  Sum/1 -> Sum1/2

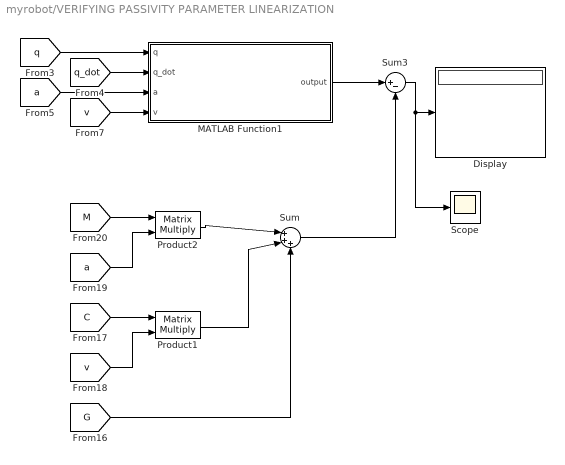
== system myrobot/VERIFYING PASSIVITY PARAMETER LINEARIZATION ==
  Display : Display
  MATLAB Function1 : MATLAB Function  TreatAsAtomicUnit=on
  Product1 : Product  Multiplication=Matrix(*)
  Product2 : Product  Multiplication=Matrix(*)
  Scope : Scope
  Sum : Sum  Inputs=|+++
  Sum3 : Sum  Inputs=|+-
  wires:
  Product1/1 -> Sum/2
  [C] -> Product1/1
  [v] -> Product1/2
  [q] -> MATLAB Function1/1(q)
  [M] -> Product2/1
  [G] -> Sum/3
  Product2/1 -> Sum/1
  [a] -> Product2/2
  [a] -> MATLAB Function1/3(a)
  Sum/1 -> Sum3/2
  MATLAB Function1/1(output) -> Sum3/1
  Sum3/1 -> Scope/1, Display/1
  [v] -> MATLAB Function1/4(v)
  [q_dot] -> MATLAB Function1/2(q_dot)

== system myrobot/TRAJECTORY GENERATION/Subsystem ==
  Constant1 : Constant  Value=0
  Constant2 : Constant  Value=0
  Constant3 : Constant  Value=0
  Constant4 : Constant
  Constant5 : Constant
  Constant6 : Constant
  Mux : Mux  Inputs=6
  Out1 : Outport
  wires:
  Mux/1 -> Out1/1
  Constant6/1 -> Mux/6
  Constant5/1 -> Mux/5
  Constant4/1 -> Mux/4
  Constant3/1 -> Mux/3
  Constant2/1 -> Mux/2
  Constant1/1 -> Mux/1

== matlab function myrobot/VERIFYING PARAMETER LINEARIZATION/MATLAB Function1 ==
  data: u output; q input; q_dot input; q_ddot input
function u = linear_parameterized(q, q_dot, q_ddot)

g = 9.81;

Y = [ q_dot(1)*q_dot(2)*sin(2*q(2)) - q_ddot(1)*(cos(2*q(2))/2 - 1/2), q_ddot(1)*sin(2*q(2)) + 2*q_dot(1)*q_dot(2)*cos(2*q(2)), q_dot(1)*((q_dot(2)*sin(2*q(2) + 2*q(3)))/2 + (q_dot(3)*sin(2*q(2) + 2*q(3)))/2) - q_ddot(1)*(cos(2*q(2) + 2*q(3))/2 - 1/2) + (q_dot(1)*q_dot(2)*sin(2*q(2) + 2*q(3)))/2 + (q_dot(1)*q_dot(3)*sin(2*q(2) + 2*q(3)))/2, q_ddot(1)*(cos(2*q(2))/2 + 1/2) - q_dot(1)*q_dot(2)*sin(2*q(2)), cos(q(2))*q_dot(2)^2 + q_ddot(2)*sin(q(2)), q_ddot(1)*sin(2*q(2) + 2*q(3)) + q_dot(1)*(q_dot(2)*cos(2*q(2) + 2*q(3)) + q_dot(3)*cos(2*q(2) + 2*q(3))) + q_dot(1)*q_dot(2)*cos(2*q(2) + 2*q(3)) + q_dot(1)*q_dot(3)*cos(2*q(2) + 2*q(3)), q_ddot(1), - sin(q(2))*q_dot(2)^2 + q_ddot(2)*cos(q(2)), q_ddot(1)*(cos(2*q(2) + 2*q(3))/2 + 1/2) - q_dot(1)*((q_dot(2)*sin(2*q(2) + 2*q(3)))/2 + (q_dot(3)*sin(2*q(2) + 2*q(3)))/2) - (q_dot(1)*q_dot(2)*sin(2*q(2) + 2*q(3)))/2 - (q_dot(1)*q_dot(3)*sin(2*q(2) + 2*q(3)))/2, q_dot(2)*(q_dot(2)*cos(q(2) + q(3)) + q_dot(3)*cos(q(2) + q(3))) + q_dot(3)*(q_dot(2)*cos(q(2) + q(3)) + q_dot(3)*cos(q(2) + q(3))) + q_ddot(2)*sin(q(2) + q(3)) + q_ddot(3)*sin(q(2) + q(3)),           0, q_ddot(2)*cos(q(2) + q(3)) - q_dot(3)*(q_dot(2)*sin(q(2) + q(3)) + q_dot(3)*sin(q(2) + q(3))) - q_dot(2)*(q_dot(2)*sin(q(2) + q(3)) + q_dot(3)*sin(q(2) + q(3))) + q_ddot(3)*cos(q(2) + q(3)),                         0,              0,              0,                       0, q_ddot(1), q_ddot(1), q_dot(1)*q_dot(2)*sin(2*q(2)) - q_ddot(1)*(cos(2*q(2))/2 - 1/2), q_ddot(1), q_dot(1)*q_dot(2)*sin(2*q(2)) - q_ddot(1)*(cos(2*q(2))/2 - 1/2), q_ddot(1), q_dot(1)*((q_dot(2)*sin(2*q(2) + 2*q(3)))/2 + (q_dot(3)*sin(2*q(2) + 2*q(3)))/2) - q_ddot(1)*(cos(2*q(2) + 2*q(3))/2 - 1/2) + (q_dot(1)*q_dot(2)*sin(2*q(2) + 2*q(3)))/2 + (q_dot(1)*q_dot(3)*sin(2*q(2) + 2*q(3)))/2, q_ddot(1), sin(q(2))*q_dot(2)^2 - q_ddot(2)*cos(q(2)), sin(q(2))*q_dot(2)^2 - q_ddot(2)*cos(q(2)), 2*q_ddot(1), q_dot(2)*(q_dot(2)*sin(q(2) + q(3)) + q_dot(3)*sin(q(2) + q(3))) + q_dot(3)*(q_dot(2)*sin(q(2) + q(3)) + q_dot(3)*sin(q(2) + q(3))) - q_ddot(2)*cos(q(2) + q(3)) - q_ddot(3)*cos(q(2) + q(3)), 2*q_ddot(1), q_dot(1)*(q_dot(2)*sin(2*q(2) + q(3)) + q_dot(3)*(sin(2*q(2) + q(3))/2 - sin(q(3))/2)) - q_ddot(1)*(cos(2*q(2) + q(3)) - cos(q(3))) - q_dot(3)*((q_dot(1)*sin(q(3)))/2 - (q_dot(1)*sin(2*q(2) + q(3)))/2) + q_dot(1)*q_dot(2)*sin(2*q(2) + q(3)), sin(q(2))*q_dot(2)^2 - q_ddot(2)*cos(q(2)), sin(q(2))*q_dot(2)^2 - q_ddot(2)*cos(q(2)), q_dot(2)*(q_dot(2)*sin(q(2) + q(3)) + q_dot(3)*sin(q(2) + q(3))) + q_dot(3)*(q_dot(2)*sin(q(2) + q(3)) + q_dot(3)*sin(q(2) + q(3))) - q_ddot(2)*cos(q(2) + q(3)) - q_ddot(3)*cos(q(2) + q(3));
                                           -(q_dot(1)^2*sin(2*q(2)))/2,                                       -q_dot(1)^2*cos(2*q(2)),                                                                                                                                                                                                                -(q_dot(1)^2*sin(2*q(2) + 2*q(3)))/2,                                            (q_dot(1)^2*sin(2*q(2)))/2,                            q_ddot(1)*sin(q(2)),                                                                                                                                                                                          -q_dot(1)^2*cos(2*q(2) + 2*q(3)),           0,                              q_ddot(1)*cos(q(2)),                                                                                                                                                                                                                 (q_dot(1)^2*sin(2*q(2) + 2*q(3)))/2,                                                                                                                                                                                                      q_ddot(1)*sin(q(2) + q(3)), q_ddot(2),                                                                                                                                                                                                      q_ddot(1)*cos(q(2) + q(3)), q_ddot(2) + q_ddot(3), -g*sin(q(2)), -g*sin(q(2)), -g*sin(q(2) + q(3)),           0,           0,                              q_ddot(2) - (q_dot(1)^2*sin(2*q(2)))/2,           0,                              q_ddot(2) - (q_dot(1)^2*sin(2*q(2)))/2,           0,                                                                                                                                                                                     q_ddot(2) + q_ddot(3) - (q_dot(1)^2*sin(2*q(2) + 2*q(3)))/2,           0,                           -q_ddot(1)*cos(q(2)),                           -q_ddot(1)*cos(q(2)),             0,                                                                                                                                                                                                     -q_ddot(1)*cos(q(2) + q(3)),             0,                                                                                                           - sin(2*q(2) + q(3))*q_dot(1)^2 + 2*q_ddot(2)*cos(q(3)) + q_ddot(3)*cos(q(3)) - q_dot(3)*sin(q(3))*(q_dot(2) + q_dot(3)) - q_dot(2)*q_dot(3)*sin(q(3)),                           -q_ddot(1)*cos(q(2)),                           -q_ddot(1)*cos(q(2)),                                                                                                                                                                                                     -q_ddot(1)*cos(q(2) + q(3));
                                                                         0,                                                                 0,                                                                                                                                                                                                                -(q_dot(1)^2*sin(2*q(2) + 2*q(3)))/2,                                                                         0,                                                  0,                                                                                                                                                                                          -q_dot(1)^2*cos(2*q(2) + 2*q(3)),           0,                                                    0,                                                                                                                                                                                                                 (q_dot(1)^2*sin(2*q(2) + 2*q(3)))/2,                                                                                                                                                                                                      q_ddot(1)*sin(q(2) + q(3)),           0,                                                                                                                                                                                                      q_ddot(1)*cos(q(2) + q(3)), q_ddot(2) + q_ddot(3),              0,              0, -g*sin(q(2) + q(3)),           0,           0,                                                                         0,           0,                                                                         0,           0,                                                                                                                                                                                     q_ddot(2) + q_ddot(3) - (q_dot(1)^2*sin(2*q(2) + 2*q(3)))/2,           0,                                                  0,                                                  0,             0,                                                                                                                                                                                                     -q_ddot(1)*cos(q(2) + q(3)),             0,                                                                                                                                                                                 (sin(q(3))/2 - sin(2*q(2) + q(3))/2)*q_dot(1)^2 + sin(q(3))*q_dot(2)^2 + q_ddot(2)*cos(q(3)),                                                  0,                                                  0,                                                                                                                                                                                                     -q_ddot(1)*cos(q(2) + q(3))];

THETA = [0.253740000000000,1.41285000000000e-07,0.0754340000000000,0.0212824000000000,-7.13886000000000e-08,2.67415000000000e-08,0.00604953000000000,0.00499483000000000,0.0104250000000000,2.13561000000000e-09,0.247523000000000,0.00274946000000000,0.0744749000000000,2.21400980000000,1.73854678600000,0.622883338500000,0.0521152000000000,0.0329527040000000,0.952024214000000,0.000192286280344500,0.371183215904572,0.0688146654633342,0.0753533118750375,0.0294165347194417,0.177120784000000,0.139083742880000,0.0598856414640000,0.0498306670800000,-0.0311344561750400,0.267839835555000,-0.167347701940840,0.159821302798087,-0.0470811354471933];


u = Y * THETA';
end
